simulink model "gm_Model"  (R2025a)
settings: Solver=FixedStepDiscrete  StartTime=0.0  StopTime=80000/fs_in  RelTol=1e-3
undefined symbols (not defined in the file or in its folder): a, b, b_fixp, beta_retanh, c, cos_omega, cos_omega_fixp, diag_count, exp_omega, exp_omega_fixp, fixp_chebacc_frac, fixp_chebacc_ws, fixp_dsp_ws, fixp_eig_frac, fixp_eig_ws, fs_in, group_size, hann_table_fixp, image_seed, image_seed_fixp, J_ROM, k, K_ROM, lap_diags, lap_main, lap_main_fi, lap_offsets, lap_offsets_fi, lap_rest, lap_rest_fi, laplacian_diags_main, laplacian_diags_offsets, laplacian_diags_rest, lut_norm_x, lut_norm_y, magnitude, n_ch, n_layer, n_px, n_px_fi, nf, norm_gain_floor, power_iters, power_norm_scaling_factor_fixp, tau, tau_fixp, theta, theta_fixp
libraries: simulink x59, hdlsllib x36, hdlstreaminglib x4, hdlmdlgenlib x1, matrix_library x1, dspvision x1
(part 2 of 8)

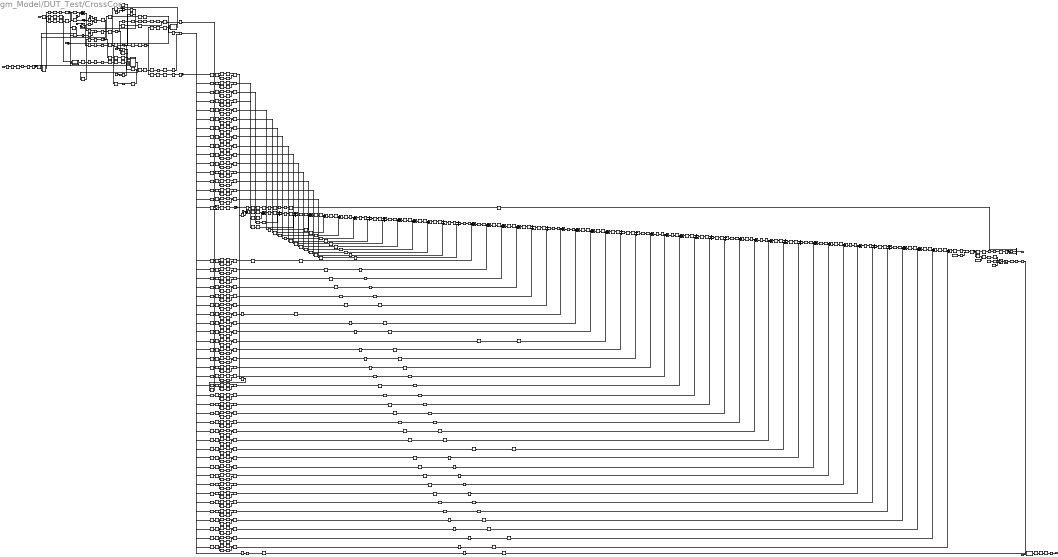
== system gm_Model/DUT_Test/CrossCor ==
  note: Sum 9 frames and reduce data rate
  valid_in : Inport  OutDataTypeStr=boolean  PortDimensions=1  SampleTime=0.0125
  data_in : Inport  Port=2  OutDataTypeStr=fixdt(1, 18, 13)  PortDimensions=[1 48]  SampleTime=0.0125
      settings: SignalType=complex
  sch_ctr_359999 : Inport  Port=3  OutDataTypeStr=fixdt(0, 19, 0)  SampleTime=3.125e-07
  sch_ctr_39999 : Inport  Port=4  OutDataTypeStr=uint16  SampleTime=3.125e-07
  AND : Logic  AllPortsSameDT=off  OutDataTypeStr=boolean  SampleTime=3.125e-07
  Bus Creator2 : BusCreator  Inputs=3
  Compare To Constant2 : simulink/Logic and Bit Operations/Compare To Constant  relop=<  const="fi(0,0,23,13,\"hex\",\"002000\")"  OutDataTypeStr=boolean
  Constant : Constant  Value=1.0001220703125  OutDataTypeStr=fixdt(0, 23, 13)  SampleTime=3.125e-07
  DataMem : RateTransition  InitialCondition=double(0)  OutPortSampleTimeOpt=Multiple of input port sample time  OutPortSampleTimeMultiple=40000
  DataMem_absorbed : Delay  DelayLength=0
  DataRT : RateTransition  InitialCondition=double(0)  OutPortSampleTimeOpt=Multiple of input port sample time  OutPortSampleTimeMultiple=9
  DataRT_outrepeat : RateTransition  Integrity=off  Deterministic=off  OutPortSampleTimeOpt=Multiple of input port sample time  OutPortSampleTimeMultiple=1/360000
  Delay{,1,7,11} (4 alike) : RateTransition  InitialCondition=double(0)  OutPortSampleTimeOpt=Multiple of input port sample time  OutPortSampleTimeMultiple=40000
  Delay1_absorbed{,1..3} (4 alike) : Delay  DelayLength=0
  Delay{2..6} (5 alike) : RateTransition  InitialCondition=double(0)  OutPortSampleTimeOpt=Multiple of input port sample time  OutPortSampleTimeMultiple=360000
  Delay2_absorbed : Delay  DelayLength=0
  Delay3_absorbed : Delay  DelayLength=0
  Delay4_absorbed : Delay  DelayLength=0
  Delay5_absorbed : Delay  DelayLength=0
  Delay6_absorbed : Delay  DelayLength=0
  Delay_Switch : Switch  Criteria=u2 ~= 0  Threshold=double(0)  OutDataTypeStr=boolean  SampleTime=3.125e-07  SaturateOnIntegerOverflow=off  InputSameDT=off
  Delay_absorbed : Delay  DelayLength=0
  Delay_absorbed1 : Delay  DelayLength=0
  Delay_absorbed2 : Delay  DelayLength=0
  Gain : Product  Inputs=**  OutDataTypeStr=fixdt(0, 23, 13)  SampleTime=3.125e-07
  Gain_const : Constant  Value=0.7071075439453125  OutDataTypeStr=fixdt(0, 18, 18)  SampleTime=3.125e-07
  HDL Counter : RateTransition  InitialCondition=double(0)  OutPortSampleTimeOpt=Multiple of input port sample time  OutPortSampleTimeMultiple=40000
  HDL Counter_absorbed : Delay  DelayLength=0
  HwModeRegister : Delay  DelayLength=double(1)  InitialCondition=0  SampleTime=3.125e-07
  HwModeRegister1 : Delay  DelayLength=double(1)  InitialCondition=0  SampleTime=3.125e-07
  Math Function1 : Math  Operator=hermitian  OutputSignalType=complex
  Max1_stage1 : MinMax  Function=max  Inputs=2
  NOT : Logic  Operator=NOT  Inputs=1  AllPortsSameDT=off  OutDataTypeStr=boolean  SampleTime=3.125e-07
  PipelineRegister : Delay  DelayLength=double(1)  InitialCondition=0  SampleTime=3.125e-07
  PipelineRegister1 : Delay  DelayLength=double(1)  InitialCondition=0  SampleTime=0.1125
  PipelineRegister2 : Delay  DelayLength=double(1)  InitialCondition=0  SampleTime=0.1125
  Real-Imag to Complex : RealImagToComplex  ConstantPart="fi(0,1,18,13,\"hex\",\"00000\")"  SampleTime=3.125e-07
  Real-Imag to Complex1 : RealImagToComplex  ConstantPart="fi(0,1,18,13,\"hex\",\"00000\")"  SampleTime=3.125e-07
  Reciprocal : Subsystem
  Row2Col_in0 : Reshape  OutputDimensionality=Column vector (2-D)
  Row2Col_in1 : Reshape  OutputDimensionality=Column vector (2-D)
  Selector : Selector  NumberOfDimensions=2  IndexOptions=Index vector (dialog),Index vector (dialog)  Indices=double(48),double(48)  OutputSizes=double(0),double(0)
  Selector1 : Selector  NumberOfDimensions=2  IndexOptions=Index vector (dialog),Index vector (dialog)  Indices=double(48),double(48)  OutputSizes=double(0),double(0)
  Selector10 : Selector  NumberOfDimensions=2  IndexOptions=Index vector (dialog),Index vector (dialog)  Indices=double(43),double(43)  OutputSizes=double(0),double(0)
  Selector11 : Selector  NumberOfDimensions=2  IndexOptions=Index vector (dialog),Index vector (dialog)  Indices=double(43),double(43)  OutputSizes=double(0),double(0)
  Selector12 : Selector  NumberOfDimensions=2  IndexOptions=Index vector (dialog),Index vector (dialog)  Indices=double(42),double(42)  OutputSizes=double(0),double(0)
  Selector13 : Selector  NumberOfDimensions=2  IndexOptions=Index vector (dialog),Index vector (dialog)  Indices=double(42),double(42)  OutputSizes=double(0),double(0)
  Selector14 : Selector  NumberOfDimensions=2  IndexOptions=Index vector (dialog),Index vector (dialog)  Indices=double(41),double(41)  OutputSizes=double(0),double(0)
  Selector15 : Selector  NumberOfDimensions=2  IndexOptions=Index vector (dialog),Index vector (dialog)  Indices=double(41),double(41)  OutputSizes=double(0),double(0)
  Selector16 : Selector  NumberOfDimensions=2  IndexOptions=Index vector (dialog),Index vector (dialog)  Indices=double(40),double(40)  OutputSizes=double(0),double(0)
  Selector17 : Selector  NumberOfDimensions=2  IndexOptions=Index vector (dialog),Index vector (dialog)  Indices=double(40),double(40)  OutputSizes=double(0),double(0)
  Selector18 : Selector  NumberOfDimensions=2  IndexOptions=Index vector (dialog),Index vector (dialog)  Indices=double(39),double(39)  OutputSizes=double(0),double(0)
  Selector19 : Selector  NumberOfDimensions=2  IndexOptions=Index vector (dialog),Index vector (dialog)  Indices=double(39),double(39)  OutputSizes=double(0),double(0)
  Selector2 : Selector  NumberOfDimensions=2  IndexOptions=Index vector (dialog),Index vector (dialog)  Indices=double(47),double(47)  OutputSizes=double(0),double(0)
  Selector20 : Selector  NumberOfDimensions=2  IndexOptions=Index vector (dialog),Index vector (dialog)  Indices=double(38),double(38)  OutputSizes=double(0),double(0)
  Selector21 : Selector  NumberOfDimensions=2  IndexOptions=Index vector (dialog),Index vector (dialog)  Indices=double(38),double(38)  OutputSizes=double(0),double(0)
  Selector22 : Selector  NumberOfDimensions=2  IndexOptions=Index vector (dialog),Index vector (dialog)  Indices=double(37),double(37)  OutputSizes=double(0),double(0)
  Selector23 : Selector  NumberOfDimensions=2  IndexOptions=Index vector (dialog),Index vector (dialog)  Indices=double(37),double(37)  OutputSizes=double(0),double(0)
  Selector24 : Selector  NumberOfDimensions=2  IndexOptions=Index vector (dialog),Index vector (dialog)  Indices=double(36),double(36)  OutputSizes=double(0),double(0)
  Selector25 : Selector  NumberOfDimensions=2  IndexOptions=Index vector (dialog),Index vector (dialog)  Indices=double(36),double(36)  OutputSizes=double(0),double(0)
  Selector26 : Selector  NumberOfDimensions=2  IndexOptions=Index vector (dialog),Index vector (dialog)  Indices=double(35),double(35)  OutputSizes=double(0),double(0)
  Selector27 : Selector  NumberOfDimensions=2  IndexOptions=Index vector (dialog),Index vector (dialog)  Indices=double(35),double(35)  OutputSizes=double(0),double(0)
  Selector28 : Selector  NumberOfDimensions=2  IndexOptions=Index vector (dialog),Index vector (dialog)  Indices=double(34),double(34)  OutputSizes=double(0),double(0)
  Selector29 : Selector  NumberOfDimensions=2  IndexOptions=Index vector (dialog),Index vector (dialog)  Indices=double(34),double(34)  OutputSizes=double(0),double(0)
  Selector3 : Selector  NumberOfDimensions=2  IndexOptions=Index vector (dialog),Index vector (dialog)  Indices=double(47),double(47)  OutputSizes=double(0),double(0)
  Selector30 : Selector  NumberOfDimensions=2  IndexOptions=Index vector (dialog),Index vector (dialog)  Indices=double(33),double(33)  OutputSizes=double(0),double(0)
  Selector31 : Selector  NumberOfDimensions=2  IndexOptions=Index vector (dialog),Index vector (dialog)  Indices=double(33),double(33)  OutputSizes=double(0),double(0)
  Selector32 : Selector  NumberOfDimensions=2  IndexOptions=Index vector (dialog),Index vector (dialog)  Indices=double(32),double(32)  OutputSizes=double(0),double(0)
  Selector33 : Selector  NumberOfDimensions=2  IndexOptions=Index vector (dialog),Index vector (dialog)  Indices=double(32),double(32)  OutputSizes=double(0),double(0)
  Selector34 : Selector  NumberOfDimensions=2  IndexOptions=Index vector (dialog),Index vector (dialog)  Indices=double(31),double(31)  OutputSizes=double(0),double(0)
  Selector35 : Selector  NumberOfDimensions=2  IndexOptions=Index vector (dialog),Index vector (dialog)  Indices=double(31),double(31)  OutputSizes=double(0),double(0)
  Selector36 : Selector  NumberOfDimensions=2  IndexOptions=Index vector (dialog),Index vector (dialog)  Indices=double(30),double(30)  OutputSizes=double(0),double(0)
  Selector37 : Selector  NumberOfDimensions=2  IndexOptions=Index vector (dialog),Index vector (dialog)  Indices=double(30),double(30)  OutputSizes=double(0),double(0)
  Selector38 : Selector  NumberOfDimensions=2  IndexOptions=Index vector (dialog),Index vector (dialog)  Indices=double(29),double(29)  OutputSizes=double(0),double(0)
  Selector39 : Selector  NumberOfDimensions=2  IndexOptions=Index vector (dialog),Index vector (dialog)  Indices=double(29),double(29)  OutputSizes=double(0),double(0)
  Selector4 : Selector  NumberOfDimensions=2  IndexOptions=Index vector (dialog),Index vector (dialog)  Indices=double(46),double(46)  OutputSizes=double(0),double(0)
  Selector40 : Selector  NumberOfDimensions=2  IndexOptions=Index vector (dialog),Index vector (dialog)  Indices=double(28),double(28)  OutputSizes=double(0),double(0)
  Selector41 : Selector  NumberOfDimensions=2  IndexOptions=Index vector (dialog),Index vector (dialog)  Indices=double(28),double(28)  OutputSizes=double(0),double(0)
  Selector42 : Selector  NumberOfDimensions=2  IndexOptions=Index vector (dialog),Index vector (dialog)  Indices=double(27),double(27)  OutputSizes=double(0),double(0)
  Selector43 : Selector  NumberOfDimensions=2  IndexOptions=Index vector (dialog),Index vector (dialog)  Indices=double(27),double(27)  OutputSizes=double(0),double(0)
  Selector44 : Selector  NumberOfDimensions=2  IndexOptions=Index vector (dialog),Index vector (dialog)  Indices=double(26),double(26)  OutputSizes=double(0),double(0)
  Selector45 : Selector  NumberOfDimensions=2  IndexOptions=Index vector (dialog),Index vector (dialog)  Indices=double(26),double(26)  OutputSizes=double(0),double(0)
  Selector46 : Selector  NumberOfDimensions=2  IndexOptions=Index vector (dialog),Index vector (dialog)  Indices=double(25),double(25)  OutputSizes=double(0),double(0)
  Selector47 : Selector  NumberOfDimensions=2  IndexOptions=Index vector (dialog),Index vector (dialog)  Indices=double(25),double(25)  OutputSizes=double(0),double(0)
  Selector48 : Selector  NumberOfDimensions=2  IndexOptions=Index vector (dialog),Index vector (dialog)  Indices=double(24),double(24)  OutputSizes=double(0),double(0)
  Selector49 : Selector  NumberOfDimensions=2  IndexOptions=Index vector (dialog),Index vector (dialog)  Indices=double(24),double(24)  OutputSizes=double(0),double(0)
  Selector5 : Selector  NumberOfDimensions=2  IndexOptions=Index vector (dialog),Index vector (dialog)  Indices=double(46),double(46)  OutputSizes=double(0),double(0)
  Selector50 : Selector  NumberOfDimensions=2  IndexOptions=Index vector (dialog),Index vector (dialog)  Indices=double(23),double(23)  OutputSizes=double(0),double(0)
  Selector51 : Selector  NumberOfDimensions=2  IndexOptions=Index vector (dialog),Index vector (dialog)  Indices=double(23),double(23)  OutputSizes=double(0),double(0)
  Selector52 : Selector  NumberOfDimensions=2  IndexOptions=Index vector (dialog),Index vector (dialog)  Indices=double(22),double(22)  OutputSizes=double(0),double(0)
  Selector53 : Selector  NumberOfDimensions=2  IndexOptions=Index vector (dialog),Index vector (dialog)  Indices=double(22),double(22)  OutputSizes=double(0),double(0)
  Selector54 : Selector  NumberOfDimensions=2  IndexOptions=Index vector (dialog),Index vector (dialog)  Indices=double(21),double(21)  OutputSizes=double(0),double(0)
  Selector55 : Selector  NumberOfDimensions=2  IndexOptions=Index vector (dialog),Index vector (dialog)  Indices=double(21),double(21)  OutputSizes=double(0),double(0)
  Selector56 : Selector  NumberOfDimensions=2  IndexOptions=Index vector (dialog),Index vector (dialog)  Indices=double(20),double(20)  OutputSizes=double(0),double(0)
  Selector57 : Selector  NumberOfDimensions=2  IndexOptions=Index vector (dialog),Index vector (dialog)  Indices=double(20),double(20)  OutputSizes=double(0),double(0)
  Selector58 : Selector  NumberOfDimensions=2  IndexOptions=Index vector (dialog),Index vector (dialog)  Indices=double(19),double(19)  OutputSizes=double(0),double(0)
  Selector59 : Selector  NumberOfDimensions=2  IndexOptions=Index vector (dialog),Index vector (dialog)  Indices=double(19),double(19)  OutputSizes=double(0),double(0)
  Selector6 : Selector  NumberOfDimensions=2  IndexOptions=Index vector (dialog),Index vector (dialog)  Indices=double(45),double(45)  OutputSizes=double(0),double(0)
  Selector60 : Selector  NumberOfDimensions=2  IndexOptions=Index vector (dialog),Index vector (dialog)  Indices=double(18),double(18)  OutputSizes=double(0),double(0)
  Selector61 : Selector  NumberOfDimensions=2  IndexOptions=Index vector (dialog),Index vector (dialog)  Indices=double(18),double(18)  OutputSizes=double(0),double(0)
  Selector62 : Selector  NumberOfDimensions=2  IndexOptions=Index vector (dialog),Index vector (dialog)  Indices=double(17),double(17)  OutputSizes=double(0),double(0)
  Selector63 : Selector  NumberOfDimensions=2  IndexOptions=Index vector (dialog),Index vector (dialog)  Indices=double(17),double(17)  OutputSizes=double(0),double(0)
  Selector64 : Selector  NumberOfDimensions=2  IndexOptions=Index vector (dialog),Index vector (dialog)  Indices=double(16),double(16)  OutputSizes=double(0),double(0)
  Selector65 : Selector  NumberOfDimensions=2  IndexOptions=Index vector (dialog),Index vector (dialog)  Indices=double(16),double(16)  OutputSizes=double(0),double(0)
  Selector66 : Selector  NumberOfDimensions=2  IndexOptions=Index vector (dialog),Index vector (dialog)  Indices=double(15),double(15)  OutputSizes=double(0),double(0)
  Selector67 : Selector  NumberOfDimensions=2  IndexOptions=Index vector (dialog),Index vector (dialog)  Indices=double(15),double(15)  OutputSizes=double(0),double(0)
  Selector68 : Selector  NumberOfDimensions=2  IndexOptions=Index vector (dialog),Index vector (dialog)  Indices=double(14),double(14)  OutputSizes=double(0),double(0)
  Selector69 : Selector  NumberOfDimensions=2  IndexOptions=Index vector (dialog),Index vector (dialog)  Indices=double(14),double(14)  OutputSizes=double(0),double(0)
  Selector7 : Selector  NumberOfDimensions=2  IndexOptions=Index vector (dialog),Index vector (dialog)  Indices=double(45),double(45)  OutputSizes=double(0),double(0)
  Selector70 : Selector  NumberOfDimensions=2  IndexOptions=Index vector (dialog),Index vector (dialog)  Indices=double(13),double(13)  OutputSizes=double(0),double(0)
  Selector71 : Selector  NumberOfDimensions=2  IndexOptions=Index vector (dialog),Index vector (dialog)  Indices=double(13),double(13)  OutputSizes=double(0),double(0)
  Selector72 : Selector  NumberOfDimensions=2  IndexOptions=Index vector (dialog),Index vector (dialog)  Indices=double(12),double(12)  OutputSizes=double(0),double(0)
  Selector73 : Selector  NumberOfDimensions=2  IndexOptions=Index vector (dialog),Index vector (dialog)  Indices=double(12),double(12)  OutputSizes=double(0),double(0)
  Selector74 : Selector  NumberOfDimensions=2  IndexOptions=Index vector (dialog),Index vector (dialog)  Indices=double(11),double(11)  OutputSizes=double(0),double(0)
  Selector75 : Selector  NumberOfDimensions=2  IndexOptions=Index vector (dialog),Index vector (dialog)  Indices=double(11),double(11)  OutputSizes=double(0),double(0)
  Selector76 : Selector  NumberOfDimensions=2  IndexOptions=Index vector (dialog),Index vector (dialog)  Indices=double(10),double(10)  OutputSizes=double(0),double(0)
  Selector77 : Selector  NumberOfDimensions=2  IndexOptions=Index vector (dialog),Index vector (dialog)  Indices=double(10),double(10)  OutputSizes=double(0),double(0)
  Selector78 : Selector  NumberOfDimensions=2  IndexOptions=Index vector (dialog),Index vector (dialog)  Indices=double(9),double(9)  OutputSizes=double(0),double(0)
  Selector79 : Selector  NumberOfDimensions=2  IndexOptions=Index vector (dialog),Index vector (dialog)  Indices=double(9),double(9)  OutputSizes=double(0),double(0)
  Selector8 : Selector  NumberOfDimensions=2  IndexOptions=Index vector (dialog),Index vector (dialog)  Indices=double(44),double(44)  OutputSizes=double(0),double(0)
  Selector80 : Selector  NumberOfDimensions=2  IndexOptions=Index vector (dialog),Index vector (dialog)  Indices=double(8),double(8)  OutputSizes=double(0),double(0)
  Selector81 : Selector  NumberOfDimensions=2  IndexOptions=Index vector (dialog),Index vector (dialog)  Indices=double(8),double(8)  OutputSizes=double(0),double(0)
  Selector82 : Selector  NumberOfDimensions=2  IndexOptions=Index vector (dialog),Index vector (dialog)  Indices=double(7),double(7)  OutputSizes=double(0),double(0)
  Selector83 : Selector  NumberOfDimensions=2  IndexOptions=Index vector (dialog),Index vector (dialog)  Indices=double(7),double(7)  OutputSizes=double(0),double(0)
  Selector84 : Selector  NumberOfDimensions=2  IndexOptions=Index vector (dialog),Index vector (dialog)  Indices=double(6),double(6)  OutputSizes=double(0),double(0)
  Selector85 : Selector  NumberOfDimensions=2  IndexOptions=Index vector (dialog),Index vector (dialog)  Indices=double(6),double(6)  OutputSizes=double(0),double(0)
  Selector86 : Selector  NumberOfDimensions=2  IndexOptions=Index vector (dialog),Index vector (dialog)  Indices=double(5),double(5)  OutputSizes=double(0),double(0)
  Selector87 : Selector  NumberOfDimensions=2  IndexOptions=Index vector (dialog),Index vector (dialog)  Indices=double(5),double(5)  OutputSizes=double(0),double(0)
  Selector88 : Selector  NumberOfDimensions=2  IndexOptions=Index vector (dialog),Index vector (dialog)  Indices=double(4),double(4)  OutputSizes=double(0),double(0)
  Selector89 : Selector  NumberOfDimensions=2  IndexOptions=Index vector (dialog),Index vector (dialog)  Indices=double(4),double(4)  OutputSizes=double(0),double(0)
  Selector9 : Selector  NumberOfDimensions=2  IndexOptions=Index vector (dialog),Index vector (dialog)  Indices=double(44),double(44)  OutputSizes=double(0),double(0)
  Selector90 : Selector  NumberOfDimensions=2  IndexOptions=Index vector (dialog),Index vector (dialog)  Indices=double(3),double(3)  OutputSizes=double(0),double(0)
  Selector91 : Selector  NumberOfDimensions=2  IndexOptions=Index vector (dialog),Index vector (dialog)  Indices=double(3),double(3)  OutputSizes=double(0),double(0)
  Selector92 : Selector  NumberOfDimensions=2  IndexOptions=Index vector (dialog),Index vector (dialog)  Indices=double(2),double(2)  OutputSizes=double(0),double(0)
  Selector93 : Selector  NumberOfDimensions=2  IndexOptions=Index vector (dialog),Index vector (dialog)  Indices=double(2),double(2)  OutputSizes=double(0),double(0)
  Selector94 : Selector  NumberOfDimensions=2  IndexOptions=Index vector (dialog),Index vector (dialog)  Indices=double(1),double(1)  OutputSizes=double(0),double(0)
  Selector95 : Selector  NumberOfDimensions=2  IndexOptions=Index vector (dialog),Index vector (dialog)  Indices=double(1),double(1)  OutputSizes=double(0),double(0)
  ValidMem_lowered : RateTransition  InitialCondition=double(0)  OutPortSampleTimeOpt=Multiple of input port sample time  OutPortSampleTimeMultiple=40000
  ValidMem_lowered_absorbed : Delay  DelayLength=0
  ValidRT : RateTransition  InitialCondition=double(0)  OutPortSampleTimeOpt=Multiple of input port sample time  OutPortSampleTimeMultiple=9
  ValidRT_outrepeat : RateTransition  Integrity=off  Deterministic=off  OutPortSampleTimeOpt=Multiple of input port sample time  OutPortSampleTimeMultiple=1/360000
  ValidResetCounter : RateTransition  InitialCondition=double(0)  OutPortSampleTimeOpt=Multiple of input port sample time  OutPortSampleTimeMultiple=40000
  ValidResetCounter_absorbed : Delay  DelayLength=0
  ValidResetDelay : RateTransition  InitialCondition=double(0)  OutPortSampleTimeOpt=Multiple of input port sample time  OutPortSampleTimeMultiple=40000
  ValidResetDelay_absorbed : Delay  DelayLength=0
  ValidSampleOR : Logic  Operator=OR  AllPortsSameDT=off  OutDataTypeStr=boolean  SampleTime=3.125e-07
  Zero : Constant  Value=0  OutDataTypeStr=fixdt(1, 18, 13)  SampleTime=3.125e-07
  Zero1 : Constant  Value=0  OutDataTypeStr=fixdt(1, 18, 13)  SampleTime=3.125e-07
  adder{,1..47} (48 alike) : Sum  OutDataTypeStr=fixdt(1, 25, 13)  AccumDataTypeStr=fixdt(1, 25, 13)  SampleTime=3.125e-07
  adder48 : Sum  OutDataTypeStr=fixdt(0, 4, 0)  AccumDataTypeStr=fixdt(0, 4, 0)  SampleTime=3.125e-07
  adder49 : Sum  OutDataTypeStr=fixdt(0, 4, 0)  AccumDataTypeStr=fixdt(0, 4, 0)  SampleTime=3.125e-07
  compare : simulink/Logic and Bit Operations/Compare To Constant  relop=>  const="fi(0,0,4,0,\"hex\",\"e\")"  OutDataTypeStr=boolean
  compare1 : simulink/Logic and Bit Operations/Compare To Constant  relop===  const="fi(0,0,4,0,\"hex\",\"8\")"  OutDataTypeStr=boolean
  compare2 : simulink/Logic and Bit Operations/Compare To Constant  relop=>  const="fi(0,0,4,0,\"hex\",\"e\")"  OutDataTypeStr=boolean
  compare3 : simulink/Logic and Bit Operations/Compare To Constant  relop===  const="fi(0,0,4,0,\"hex\",\"8\")"  OutDataTypeStr=boolean
  const : Constant  Value=0  VectorParams1D=off  OutDataTypeStr=fixdt(0, 23, 13)  SampleTime=3.125e-07
  countFrom : Constant  Value=0  VectorParams1D=off  OutDataTypeStr=fixdt(0, 4, 0)  SampleTime=3.125e-07
  countFrom1 : Constant  Value=0  VectorParams1D=off  OutDataTypeStr=fixdt(0, 4, 0)  SampleTime=3.125e-07
  cplx2reim{,1..47} (48 alike) : ComplexToRealImag  Output=Real  SampleTime=3.125e-07
  cplx2reim{48..95} (48 alike) : ComplexToRealImag  SampleTime=3.125e-07
  crp_out_delay{,1..11} (12 alike) : Delay  DelayLength=double(1)  InitialCondition=0  SampleTime=3.125e-07
  default_value : Constant  Value=fi(1,0,23,13)  OutDataTypeStr=fixdt(0, 23, 13)  SampleTime=3.125e-07
  delayMatch : Delay  DelayLength=double(40000)  InitialCondition=0  SampleTime=3.125e-07
  delayMatch1 : Delay  DelayLength=double(8)  InitialCondition=0  SampleTime=0.0125
  delayMatch2 : Delay  DelayLength=double(8)  InitialCondition=0  SampleTime=0.0125
  delayMatch3 : Delay  DelayLength=double(360000)  InitialCondition=0  SampleTime=3.125e-07
  delayMatch4 : Delay  DelayLength=double(360000)  InitialCondition=0  SampleTime=3.125e-07
  dtc{,1..47} (48 alike) : DataTypeConversion  OutDataTypeStr=fixdt(0, 23, 13)  SampleTime=3.125e-07  SaturateOnIntegerOverflow=off  RndMeth=Floor
  dtc48 : hdlmdlgenlib/Buffer
  in0_repeat : RateTransition  Integrity=off  Deterministic=off  OutPortSampleTimeOpt=Multiple of input port sample time  OutPortSampleTimeMultiple=1/40000
  in0_repeat1 : RateTransition  Integrity=off  Deterministic=off  OutPortSampleTimeOpt=Multiple of input port sample time  OutPortSampleTimeMultiple=1/40000
  in0_repeat2 : RateTransition  Integrity=off  Deterministic=off  OutPortSampleTimeOpt=Multiple of input port sample time  OutPortSampleTimeMultiple=1/360000
  in0_repeat3 : RateTransition  Integrity=off  Deterministic=off  OutPortSampleTimeOpt=Multiple of input port sample time  OutPortSampleTimeMultiple=1/40000
  in1_repeat : RateTransition  Integrity=off  Deterministic=off  OutPortSampleTimeOpt=Multiple of input port sample time  OutPortSampleTimeMultiple=1/40000
  in1_repeat1 : RateTransition  Integrity=off  Deterministic=off  OutPortSampleTimeOpt=Multiple of input port sample time  OutPortSampleTimeMultiple=1/360000
  in1_repeat2 : RateTransition  Integrity=off  Deterministic=off  OutPortSampleTimeOpt=Multiple of input port sample time  OutPortSampleTimeMultiple=1/40000
  in1_repeat3 : RateTransition  Integrity=off  Deterministic=off  OutPortSampleTimeOpt=Multiple of input port sample time  OutPortSampleTimeMultiple=1/40000
  in2_repeat : RateTransition  Integrity=off  Deterministic=off  OutPortSampleTimeOpt=Multiple of input port sample time  OutPortSampleTimeMultiple=1/40000
  in2_repeat1 : RateTransition  Integrity=off  Deterministic=off  OutPortSampleTimeOpt=Multiple of input port sample time  OutPortSampleTimeMultiple=1/360000
  in2_repeat2 : RateTransition  Integrity=off  Deterministic=off  OutPortSampleTimeOpt=Multiple of input port sample time  OutPortSampleTimeMultiple=1/40000
  in2_repeat3 : RateTransition  Integrity=off  Deterministic=off  OutPortSampleTimeOpt=Multiple of input port sample time  OutPortSampleTimeMultiple=1/40000
  in3_repeat : RateTransition  Integrity=off  Deterministic=off  OutPortSampleTimeOpt=Multiple of input port sample time  OutPortSampleTimeMultiple=1/40000
  in3_repeat1 : RateTransition  Integrity=off  Deterministic=off  OutPortSampleTimeOpt=Multiple of input port sample time  OutPortSampleTimeMultiple=1/360000
  in3_repeat2 : RateTransition  Integrity=off  Deterministic=off  OutPortSampleTimeOpt=Multiple of input port sample time  OutPortSampleTimeMultiple=1/40000
  in4_repeat : RateTransition  Integrity=off  Deterministic=off  OutPortSampleTimeOpt=Multiple of input port sample time  OutPortSampleTimeMultiple=1/40000
  in4_repeat1 : RateTransition  Integrity=off  Deterministic=off  OutPortSampleTimeOpt=Multiple of input port sample time  OutPortSampleTimeMultiple=1/40000
  in5_repeat : RateTransition  Integrity=off  Deterministic=off  OutPortSampleTimeOpt=Multiple of input port sample time  OutPortSampleTimeMultiple=1/40000
  or : Logic  Operator=OR  AllPortsSameDT=off  OutDataTypeStr=boolean  SampleTime=3.125e-07
  or1 : Logic  Operator=OR  AllPortsSameDT=off  OutDataTypeStr=boolean  SampleTime=3.125e-07
  rd_{0..4,6,8,10,12,14,16,18,20,22,24,26,28,30,32,34,36,38,40,42,44,46,48,50,52,54,56,58,60,62,64,66,68,70,72,74,76,78,80,82,84,86,88,90,92,94,96..98,101..102,110..112,121,131,141,210..212,310,411,510..511,610..612,710,810,910} (74 alike) : Delay  DelayLength=double(1)  InitialCondition=0  SampleTime=3.125e-07
  rd_01 : Delay  DelayLength=double(1)  InitialCondition=0  SampleTime=3.125e-07
  rd_02 : Delay  DelayLength=double(1)  InitialCondition=0  SampleTime=3.125e-07
  rd_03 : Delay  DelayLength=double(1)  InitialCondition=0  SampleTime=3.125e-07
  rd_04 : Delay  DelayLength=double(1)  InitialCondition=0  SampleTime=3.125e-07
  rd_103 : Delay  DelayLength=double(4)  InitialCondition=0  SampleTime=3.125e-07
  rd_11 : Delay  DelayLength=double(5)  InitialCondition=0  SampleTime=3.125e-07
  rd_13 : Delay  DelayLength=double(6)  InitialCondition=0  SampleTime=3.125e-07
  rd_15 : Delay  DelayLength=double(7)  InitialCondition=0  SampleTime=3.125e-07
  rd_17 : Delay  DelayLength=double(8)  InitialCondition=0  SampleTime=3.125e-07
  rd_19 : Delay  DelayLength=double(9)  InitialCondition=0  SampleTime=3.125e-07
  rd_21 : Delay  DelayLength=double(10)  InitialCondition=0  SampleTime=3.125e-07
  rd_23 : Delay  DelayLength=double(11)  InitialCondition=0  SampleTime=3.125e-07
  rd_25 : Delay  DelayLength=double(12)  InitialCondition=0  SampleTime=3.125e-07
  rd_27 : Delay  DelayLength=double(13)  InitialCondition=0  SampleTime=3.125e-07
  rd_29 : Delay  DelayLength=double(14)  InitialCondition=0  SampleTime=3.125e-07
  rd_31 : Delay  DelayLength=double(15)  InitialCondition=0  SampleTime=3.125e-07
  rd_{5,311,410,712} (4 alike) : Delay  DelayLength=double(2)  InitialCondition=0  SampleTime=3.125e-07
  rd_33 : Delay  DelayLength=double(16)  InitialCondition=0  SampleTime=3.125e-07
  rd_35 : Delay  DelayLength=double(17)  InitialCondition=0  SampleTime=3.125e-07
  rd_37 : Delay  DelayLength=double(18)  InitialCondition=0  SampleTime=3.125e-07
  rd_39 : Delay  DelayLength=double(19)  InitialCondition=0  SampleTime=3.125e-07
  rd_41 : Delay  DelayLength=double(20)  InitialCondition=0  SampleTime=3.125e-07
  rd_43 : Delay  DelayLength=double(21)  InitialCondition=0  SampleTime=3.125e-07
  rd_45 : Delay  DelayLength=double(22)  InitialCondition=0  SampleTime=3.125e-07
  rd_47 : Delay  DelayLength=double(23)  InitialCondition=0  SampleTime=3.125e-07
  rd_49 : Delay  DelayLength=double(24)  InitialCondition=0  SampleTime=3.125e-07
  rd_51 : Delay  DelayLength=double(25)  InitialCondition=0  SampleTime=3.125e-07
  rd_53 : Delay  DelayLength=double(26)  InitialCondition=0  SampleTime=3.125e-07
  rd_55 : Delay  DelayLength=double(27)  InitialCondition=0  SampleTime=3.125e-07
  rd_57 : Delay  DelayLength=double(28)  InitialCondition=0  SampleTime=3.125e-07
  rd_59 : Delay  DelayLength=double(29)  InitialCondition=0  SampleTime=3.125e-07
  rd_61 : Delay  DelayLength=double(30)  InitialCondition=0  SampleTime=3.125e-07
  rd_63 : Delay  DelayLength=double(31)  InitialCondition=0  SampleTime=3.125e-07
  rd_65 : Delay  DelayLength=double(32)  InitialCondition=0  SampleTime=3.125e-07
  rd_67 : Delay  DelayLength=double(33)  InitialCondition=0  SampleTime=3.125e-07
  rd_69 : Delay  DelayLength=double(34)  InitialCondition=0  SampleTime=3.125e-07
  rd_7 : Delay  DelayLength=double(3)  InitialCondition=0  SampleTime=3.125e-07
  rd_71 : Delay  DelayLength=double(35)  InitialCondition=0  SampleTime=3.125e-07
  rd_711 : Delay  DelayLength=double(3)  InitialCondition=0  SampleTime=3.125e-07
  rd_73 : Delay  DelayLength=double(36)  InitialCondition=0  SampleTime=3.125e-07
  rd_75 : Delay  DelayLength=double(37)  InitialCondition=0  SampleTime=3.125e-07
  rd_77 : Delay  DelayLength=double(38)  InitialCondition=0  SampleTime=3.125e-07
  rd_79 : Delay  DelayLength=double(39)  InitialCondition=0  SampleTime=3.125e-07
  rd_81 : Delay  DelayLength=double(40)  InitialCondition=0  SampleTime=3.125e-07
  rd_811 : Delay  DelayLength=double(3)  InitialCondition=0  SampleTime=3.125e-07
  rd_83 : Delay  DelayLength=double(41)  InitialCondition=0  SampleTime=3.125e-07
  rd_85 : Delay  DelayLength=double(42)  InitialCondition=0  SampleTime=3.125e-07
  rd_87 : Delay  DelayLength=double(43)  InitialCondition=0  SampleTime=3.125e-07
  rd_89 : Delay  DelayLength=double(44)  InitialCondition=0  SampleTime=3.125e-07
  rd_9 : Delay  DelayLength=double(4)  InitialCondition=0  SampleTime=3.125e-07
  rd_91 : Delay  DelayLength=double(45)  InitialCondition=0  SampleTime=3.125e-07
  rd_93 : Delay  DelayLength=double(46)  InitialCondition=0  SampleTime=3.125e-07
  rd_95 : Delay  DelayLength=double(47)  InitialCondition=0  SampleTime=3.125e-07
  rd_99 : Delay  DelayLength=double(51)  InitialCondition=0  SampleTime=3.125e-07
  reim2cplx{,1..47} (48 alike) : RealImagToComplex  ConstantPart="fi(0,1,18,13,\"hex\",\"00000\")"  SampleTime=3.125e-07
  reshape_mmulResult : Reshape  OutputDimensionality=Customize  OutputDimensions=[48,48]
  select_indices0 : Selector  InputPortWidth=48  IndexOptions=Index vector (dialog)  Indices=double([1;2;3;4;5;6;7;8;9;10;11;12;13;14;15;16;17;18;19;20;21;22;23;24;25;26;27;28;29;30;31;32;33;34;35;36;37;38;39;40;41;42;43;44;45;46;47;48;1;2;3;4;5;6;7;8;9;10;11;12;13;14;15;16;17;18;19;20;21;22;23;24;25;26;27;28;29;30;31;32;33;34;35;36;37;38;39;40;41;42;43;44;45;46;47;48;1;2;3;4;5;6;7;8;9;10;11;12;13;14;15;16;17;18;19;20;21;22;23;24;25;26;27;28;29;30;31;32;33;34;35;36;37;38;39;40;41;42;43;44;45;46;47;48;1;2;3;4;5;6;7;8;9;10;11;12;13;14;15;16;17;18;19;20;21;22;23;24;25;26;27;28;29;30;31;32;33;34;35;36;37;38;39;40;41;42;43;44;45;46;47;48;1;2;3;4;5;6;7;8;9;10;11;12;13;14;15;16;17;18;19;20;21;22;23;24;25;26;27;28;29;30;31;32;33;34;35;36;37;38;39;40;41;42;43;44;45;46;47;48;1;2;3;4;5;6;7;8;9;10;11;12;13;14;15;16;17;18;19;20;21;22;23;24;25;26;27;28;29;30;31;32;33;34;35;36;37;38;39;40;41;42;43;44;45;46;47;48;1;2;3;4;5;6;7;8;9;10;11;12;13;14;15;16;17;18;19;20;21;22;23;24;25;26;27;28;29;30;31;32;33;34;35;36;37;38;39;40;41;42;43;44;45;46;47;48;1;2;3;4;5;6;7;8;9;10;11;12;13;14;15;16;17;18;19;20;21;22;23;24;25;26;27;28;29;30;31;32;33;34;35;36;37;38;39;40;41;42;43;44;45;46;47;48;1;2;3;4;5;6;7;8;9;10;11;12;13;14;15;16;17;18;19;20;21;22;23;24;25;26;27;28;29;30;31;32;33;34;35;36;37;38;39;40;41;42;43;44;45;46;47;48;1;2;3;4;5;6;7;8;9;10;11;12;13;14;15;16;17;18;19;20;21;22;23;24;25;26;27;28;29;30;31;32;33;34;35;36;37;38;39;40;41;42;43;44;45;46;47;48;1;2;3;4;5;6;7;8;9;10;11;12;13;14;15;16;17;18;19;20;21;22;23;24;25;26;27;28;29;30;31;32;33;34;35;36;37;38;39;40;41;42;43;44;45;46;47;48;1;2;3;4;5;6;7;8;9;10;11;12;13;14;15;16;17;18;19;20;21;22;23;24;25;26;27;28;29;30;31;32;33;34;35;36;37;38;39;40;41;42;43;44;45;46;47;48;1;2;3;4;5;6;7;8;9;10;11;12;13;14;15;16;17;18;19;20;21;22;23;24;25;26;27;28;29;30;31;32;33;34;35;36;37;38;39;40;41;42;43;44;45;46;47;48;1;2;3;4;5;6;7;8;9;10;11;12;13;14;15;16;17;18;19;20;21;22;23;24;25;26;27;28;29;30;31;32;33;34;35;36;37;38;39;40;41;42;43;44;45;46;47;48;1;2;3;4;5;6;7;8;9;10;11;12;13;14;15;16;17;18;19;20;21;22;23;24;25;26;27;28;29;30;31;32;33;34;35;36;37;38;39;40;41;42;43;44;45;46;47;48;1;2;3;4;5;6;7;8;9;10;11;12;13;14;15;16;17;18;19;20;21;22;23;24;25;26;27;28;29;30;31;32;33;34;35;36;37;38;39;40;41;42;43;44;45;46;47;48;1;2;3;4;5;6;7;8;9;10;11;12;13;14;15;16;17;18;19;20;21;22;23;24;25;26;27;28;29;30;31;32;33;34;35;36;37;38;39;40;41;42;43;44;45;46;47;48;1;2;3;4;5;6;7;8;9;10;11;12;13;14;15;16;17;18;19;20;21;22;23;24;25;26;27;28;29;30;31;32;33;34;35;36;37;38;39;40;41;42;43;44;45;46;47;48;1;2;3;4;5;6;7;8;9;10;11;12;13;14;15;16;17;18;19;20;21;22;23;24;25;26;27;28;29;30;31;32;33;34;35;36;37;38;39;40;41;42;43;44;45;46;47;48;1;2;3;4;5;6;7;8;9;10;11;12;13;14;15;16;17;18;19;20;21;22;23;24;25;26;27;28;29;30;31;32;33;34;35;36;37;38;39;40;41;42;43;44;45;46;47;48;1;2;3;4;5;6;7;8;9;10;11;12;13;14;15;16;17;18;19;20;21;22;23;24;25;26;27;28;29;30;31;32;33;34;35;36;37;38;39;40;41;42;43;44;45;46;47;48;1;2;3;4;5;6;7;8;9;10;11;12;13;14;15;16;17;18;19;20;21;22;23;24;25;26;27;28;29;30;31;32;33;34;35;36;37;38;39;40;41;42;43;44;45;46;47;48;1;2;3;4;5;6;7;8;9;10;11;12;13;14;15;16;17;18;19;20;21;22;23;24;25;26;27;28;29;30;31;32;33;34;35;36;37;38;39;40;41;42;43;44;45;46;47;48;1;2;3;4;5;6;7;8;9;10;11;12;13;14;15;16;17;18;19;20;21;22;23;24;25;26;27;28;29;30;31;32;33;34;35;36;37;38;39;40;41;42;43;44;45;46;47;48;1;2;3;4;5;6;7;8;9;10;11;12;13;14;15;16;17;18;19;20;21;22;23;24;25;26;27;28;29;30;31;32;33;34;35;36;37;38;39;40;41;42;43;44;45;46;47;48;1;2;3;4;5;6;7;8;9;10;11;12;13;14;15;16;17;18;19;20;21;22;23;24;25;26;27;28;29;30;31;32;33;34;35;36;37;38;39;40;41;42;43;44;45;46;47;48;1;2;3;4;5;6;7;8;9;10;11;12;13;14;15;16;17;18;19;20;21;22;23;24;25;26;27;28;29;30;31;32;33;34;35;36;37;38;39;40;41;42;43;44;45;46;47;48;1;2;3;4;5;6;7;8;9;10;11;12;13;14;15;16;17;18;19;20;21;22;23;24;25;26;27;28;29;30;31;32;33;34;35;36;37;38;39;40;41;42;43;44;45;46;47;48;1;2;3;4;5;6;7;8;9;10;11;12;13;14;15;16;17;18;19;20;21;22;23;24;25;26;27;28;29;30;31;32;33;34;35;36;37;38;39;40;41;42;43;44;45;46;47;48;1;2;3;4;5;6;7;8;9;10;11;12;13;14;15;16;17;18;19;20;21;22;23;24;25;26;27;28;29;30;31 ...(+2481 chars)])  OutputSizes=1
  select_indices1 : Selector  InputPortWidth=48  IndexOptions=Index vector (dialog)  Indices=double([1;1;1;1;1;1;1;1;1;1;1;1;1;1;1;1;1;1;1;1;1;1;1;1;1;1;1;1;1;1;1;1;1;1;1;1;1;1;1;1;1;1;1;1;1;1;1;1;2;2;2;2;2;2;2;2;2;2;2;2;2;2;2;2;2;2;2;2;2;2;2;2;2;2;2;2;2;2;2;2;2;2;2;2;2;2;2;2;2;2;2;2;2;2;2;2;3;3;3;3;3;3;3;3;3;3;3;3;3;3;3;3;3;3;3;3;3;3;3;3;3;3;3;3;3;3;3;3;3;3;3;3;3;3;3;3;3;3;3;3;3;3;3;3;4;4;4;4;4;4;4;4;4;4;4;4;4;4;4;4;4;4;4;4;4;4;4;4;4;4;4;4;4;4;4;4;4;4;4;4;4;4;4;4;4;4;4;4;4;4;4;4;5;5;5;5;5;5;5;5;5;5;5;5;5;5;5;5;5;5;5;5;5;5;5;5;5;5;5;5;5;5;5;5;5;5;5;5;5;5;5;5;5;5;5;5;5;5;5;5;6;6;6;6;6;6;6;6;6;6;6;6;6;6;6;6;6;6;6;6;6;6;6;6;6;6;6;6;6;6;6;6;6;6;6;6;6;6;6;6;6;6;6;6;6;6;6;6;7;7;7;7;7;7;7;7;7;7;7;7;7;7;7;7;7;7;7;7;7;7;7;7;7;7;7;7;7;7;7;7;7;7;7;7;7;7;7;7;7;7;7;7;7;7;7;7;8;8;8;8;8;8;8;8;8;8;8;8;8;8;8;8;8;8;8;8;8;8;8;8;8;8;8;8;8;8;8;8;8;8;8;8;8;8;8;8;8;8;8;8;8;8;8;8;9;9;9;9;9;9;9;9;9;9;9;9;9;9;9;9;9;9;9;9;9;9;9;9;9;9;9;9;9;9;9;9;9;9;9;9;9;9;9;9;9;9;9;9;9;9;9;9;10;10;10;10;10;10;10;10;10;10;10;10;10;10;10;10;10;10;10;10;10;10;10;10;10;10;10;10;10;10;10;10;10;10;10;10;10;10;10;10;10;10;10;10;10;10;10;10;11;11;11;11;11;11;11;11;11;11;11;11;11;11;11;11;11;11;11;11;11;11;11;11;11;11;11;11;11;11;11;11;11;11;11;11;11;11;11;11;11;11;11;11;11;11;11;11;12;12;12;12;12;12;12;12;12;12;12;12;12;12;12;12;12;12;12;12;12;12;12;12;12;12;12;12;12;12;12;12;12;12;12;12;12;12;12;12;12;12;12;12;12;12;12;12;13;13;13;13;13;13;13;13;13;13;13;13;13;13;13;13;13;13;13;13;13;13;13;13;13;13;13;13;13;13;13;13;13;13;13;13;13;13;13;13;13;13;13;13;13;13;13;13;14;14;14;14;14;14;14;14;14;14;14;14;14;14;14;14;14;14;14;14;14;14;14;14;14;14;14;14;14;14;14;14;14;14;14;14;14;14;14;14;14;14;14;14;14;14;14;14;15;15;15;15;15;15;15;15;15;15;15;15;15;15;15;15;15;15;15;15;15;15;15;15;15;15;15;15;15;15;15;15;15;15;15;15;15;15;15;15;15;15;15;15;15;15;15;15;16;16;16;16;16;16;16;16;16;16;16;16;16;16;16;16;16;16;16;16;16;16;16;16;16;16;16;16;16;16;16;16;16;16;16;16;16;16;16;16;16;16;16;16;16;16;16;16;17;17;17;17;17;17;17;17;17;17;17;17;17;17;17;17;17;17;17;17;17;17;17;17;17;17;17;17;17;17;17;17;17;17;17;17;17;17;17;17;17;17;17;17;17;17;17;17;18;18;18;18;18;18;18;18;18;18;18;18;18;18;18;18;18;18;18;18;18;18;18;18;18;18;18;18;18;18;18;18;18;18;18;18;18;18;18;18;18;18;18;18;18;18;18;18;19;19;19;19;19;19;19;19;19;19;19;19;19;19;19;19;19;19;19;19;19;19;19;19;19;19;19;19;19;19;19;19;19;19;19;19;19;19;19;19;19;19;19;19;19;19;19;19;20;20;20;20;20;20;20;20;20;20;20;20;20;20;20;20;20;20;20;20;20;20;20;20;20;20;20;20;20;20;20;20;20;20;20;20;20;20;20;20;20;20;20;20;20;20;20;20;21;21;21;21;21;21;21;21;21;21;21;21;21;21;21;21;21;21;21;21;21;21;21;21;21;21;21;21;21;21;21;21;21;21;21;21;21;21;21;21;21;21;21;21;21;21;21;21;22;22;22;22;22;22;22;22;22;22;22;22;22;22;22;22;22;22;22;22;22;22;22;22;22;22;22;22;22;22;22;22;22;22;22;22;22;22;22;22;22;22;22;22;22;22;22;22;23;23;23;23;23;23;23;23;23;23;23;23;23;23;23;23;23;23;23;23;23;23;23;23;23;23;23;23;23;23;23;23;23;23;23;23;23;23;23;23;23;23;23;23;23;23;23;23;24;24;24;24;24;24;24;24;24;24;24;24;24;24;24;24;24;24;24;24;24;24;24;24;24;24;24;24;24;24;24;24;24;24;24;24;24;24;24;24;24;24;24;24;24;24;24;24;25;25;25;25;25;25;25;25;25;25;25;25;25;25;25;25;25;25;25;25;25;25;25;25;25;25;25;25;25;25;25;25;25;25;25;25;25;25;25;25;25;25;25;25;25;25;25;25;26;26;26;26;26;26;26;26;26;26;26;26;26;26;26;26;26;26;26;26;26;26;26;26;26;26;26;26;26;26;26;26;26;26;26;26;26;26;26;26;26;26;26;26;26;26;26;26;27;27;27;27;27;27;27;27;27;27;27;27;27;27;27;27;27;27;27;27;27;27;27;27;27;27;27;27;27;27;27;27;27;27;27;27;27;27;27;27;27;27;27;27;27;27;27;27;28;28;28;28;28;28;28;28;28;28;28;28;28;28;28;28;28;28;28;28;28;28;28;28;28;28;28;28;28;28;28;28;28;28;28;28;28;28;28;28;28;28;28;28;28;28;28;28;29;29;29;29;29;29;29;29;29;29;29;29;29;29;29;29;29;29;29;29;29;29;29;29;29;29;29;29;29;29;29;29;29;29;29;29;29;29;29;29;29;29;29;29;29;29;29;29;30;30;30;30;30;30;30;30;30;30;30;30;30;30;30;30;30;30;30;30;30;30;30;30;30;30;30;30;30;30;30;30;30;30;30;30;30;30;30;30;30;30;30;30;30;30;30;30;31;31;31;31;31;31;31;31;31;31;31;31;31;31;31;31;31;31;31;31;31;31;31;31;31;31;31;31;31;31;31;31;31;31;31;31;31 ...(+2481 chars)])  OutputSizes=1
  select_signal : Constant  Value=double(1)  OutDataTypeStr=boolean  SampleTime=3.125e-07
  step_value : Constant  VectorParams1D=off  OutDataTypeStr=fixdt(0, 4, 0)  SampleTime=3.125e-07
  step_value1 : Constant  VectorParams1D=off  OutDataTypeStr=fixdt(0, 4, 0)  SampleTime=3.125e-07
  streaming_partition_streamed : Subsystem
  streaming_partition_streamed1 : Subsystem
  streaming_partition_streamed2 : Subsystem
  streaming_partition_streamed3 : Subsystem
  switch : Switch  Criteria=u2 ~= 0  Threshold="fi(0,0,1,0,\"hex\",\"0\")"  OutDataTypeStr=fixdt(0, 4, 0)  SampleTime=3.125e-07  SaturateOnIntegerOverflow=off  InputSameDT=off
  switch1 : Switch  Criteria=u2 ~= 0  Threshold="fi(0,0,1,0,\"hex\",\"0\")"  OutDataTypeStr=fixdt(0, 4, 0)  SampleTime=3.125e-07  SaturateOnIntegerOverflow=off  InputSameDT=off
  switchEnable : MultiPortSwitch  DataPortOrder=Zero-based contiguous  Inputs=2  DiagnosticForDefault=None  zeroidx=on  OutDataTypeStr=fixdt(0, 4, 0)  SampleTime=3.125e-07  SaturateOnIntegerOverflow=off  InputSameDT=off
  t{,2,5,8,11,14,17,20,23,26,29,32,35,38,41,44,47,50,53,56,59,62,65,68,71,74,77,80,83,86,89,92,95,98,101,104,107,110,113,116,119,122,125,128,131,134,137,140,143,146..147,149..150} (53 alike) : Reshape  OutputDimensionality=Column vector (2-D)
  t{1,3..4,6..7,9..10,12..13,15..16,18..19,21..22,24..25,27..28,30..31,33..34,36..37,39..40,42..43,45..46,48..49,51..52,54..55,57..58,60..61,63..64,66..67,69..70,72..73,75..76,78..79,81..82,84..85,87..88,90..91,93..94,96..97,99..100,102..103,105..106,108..109,111..112,114..115,117..118,120..121,123..124,126..127,129..130,132..133,135..136,138..139,141..142,144..145,148,151} (99 alike) : Reshape  OutputDimensionality=Customize  OutputDimensions=[48,48]
  zero_protection : Switch  Criteria=u2 ~= 0  Threshold=double(0)  OutDataTypeStr=fixdt(0, 23, 13)  SampleTime=3.125e-07  SaturateOnIntegerOverflow=off  InputSameDT=off
  status : Outport
  data_out : Outport  Port=2  SampleTime=0.1125
  wires:
  adder29/1 -> dtc29/1
  rd_26/1 -> adder34/1
  cplx2reim92/1 -> t138/1
  rd_411/1 -> t150/1
  dtc14/1 -> rd_68/1
  adder3/1 -> dtc3/1
  Selector/1 -> reim2cplx/2
  t8/1 -> cplx2reim49/1
  Gain/1 -> PipelineRegister/1
  Selector89/1 -> reim2cplx44/1
  reim2cplx7/1 -> cplx2reim7/1
  reim2cplx17/1 -> cplx2reim17/1
  rd_1/1 -> adder48/1
  cplx2reim82/1 -> t108/1
  t30/1 -> Selector19/1
  adder45/1 -> dtc45/1
  HwModeRegister1/1 -> Gain/2
  DataRT_outrepeat/1 -> rd_01/1
  cplx2reim82/2 -> t109/1
  Selector17/1 -> reim2cplx8/1
  Delay2_absorbed/1 -> data_out/1
  adder33/1 -> dtc33/1
  cplx2reim90/2 -> t133/1
  select_indices1/1 -> Row2Col_in1/1
  cplx2reim50/1 -> t12/1
  rd_111/1 -> Math Function1/1
  Selector64/1 -> reim2cplx32/2
  t51/1 -> Selector33/1
  rd_18/1 -> adder38/1
  streaming_partition_streamed/1(out0) -> t1/1
  t143/1 -> cplx2reim94/1
  cplx2reim23/1 -> rd_49/1
  t63/1 -> Selector41/1
  rd_910/1 -> Delay_Switch/2
  cplx2reim80/2 -> t103/1
  Real-Imag to Complex1/1 -> streaming_partition_streamed2/6(in5)
  Selector41/1 -> reim2cplx20/1
  t101/1 -> cplx2reim80/1
  cplx2reim38/1 -> rd_19/1
  DataRT/1 -> PipelineRegister1/1
  t102/1 -> Selector67/1
  ValidRT/1 -> PipelineRegister2/1
  cplx2reim86/2 -> t121/1
  t38/1 -> cplx2reim59/1
  rd_42/1 -> adder26/1
  rd_112/1 -> NOT/1
  cplx2reim61/2 -> t46/1
  HwModeRegister/1 -> Gain/1
  rd_141/1 -> or1/2
  t9/1 -> Selector5/1
  rd_3/1 -> adder46/2
  reshape_mmulResult/1 -> crp_out_delay6/1
  t5/1 -> cplx2reim48/1
  dtc32/1 -> rd_32/1
  rd_64/1 -> adder15/1
  t48/1 -> Selector31/1
  adder15/1 -> dtc15/1
  Max1_stage1/1 -> dtc48/1
  compare2/1 -> rd_141/1
  cplx2reim41/1 -> rd_13/1
  t136/1 -> Selector88/1
  rd_511/1 -> compare3/1
  t105/1 -> Selector69/1
  rd_22/1 -> adder36/1
  Selector63/1 -> reim2cplx31/1
  Selector94/1 -> reim2cplx47/2
  reim2cplx47/1 -> cplx2reim47/1
  rd_510/1 -> or/1
  t92/1 -> cplx2reim77/1
  crp_out_delay7/1 -> Delay7/1
  cplx2reim67/2 -> t64/1
  adder17/1 -> dtc17/1
  t86/1 -> cplx2reim75/1
  switchEnable/1 -> crp_out_delay8/1
  dtc5/1 -> rd_86/1
  rd_74/1 -> adder10/1
  or1/1 -> crp_out_delay9/1
  ValidMem_lowered/1 -> ValidMem_lowered_absorbed/1
  dtc47/1 -> rd_2/1
  Delay1/1 -> Delay1_absorbed/1
  rd_44/1 -> adder25/1
  rd_811/1 -> ValidSampleOR/2
  crp_out_delay3/1 -> ValidResetCounter/1
  cplx2reim91/1 -> t135/1
  adder11/1 -> dtc11/1
  PipelineRegister2/1 -> ValidRT_outrepeat/1
  in0_repeat3/1 -> rd_1/1, rd_610/1, rd_02/1
  Selector68/1 -> reim2cplx34/2
  zero_protection/1 -> Reciprocal/1(In1)
  dtc28/1 -> rd_40/1
  reim2cplx33/1 -> cplx2reim33/1
  ValidMem_lowered_absorbed/1 -> delayMatch2/1, in2_repeat3/1
  cplx2reim57/1 -> t33/1
  t17/1 -> cplx2reim52/1
  reim2cplx32/1 -> cplx2reim32/1
  rd_82/1 -> adder6/1
  t68/1 -> cplx2reim69/1
  t138/1 -> Selector91/1
  dtc34/1 -> rd_28/1
  Selector30/1 -> reim2cplx15/2
  default_value/1 -> zero_protection/3
  t36/1 -> Selector23/1
  rd_70/1 -> adder12/1
  dtc31/1 -> rd_34/1
  cplx2reim11/1 -> rd_73/1
  t24/1 -> Selector15/1
  sch_ctr_359999/1 -> streaming_partition_streamed/3(enb_counter)
  HDL Counter/1 -> HDL Counter_absorbed/1
  Selector51/1 -> reim2cplx25/1
  t57/1 -> Selector37/1
  cplx2reim69/2 -> t70/1
  Selector7/1 -> reim2cplx3/1
  t81/1 -> Selector53/1
  Bus Creator2/1 -> status/1
  cplx2reim59/2 -> t40/1
  rd_110/1 -> t146/1
  rd_612/1 -> ValidSampleOR/1
  t144/1 -> Selector95/1
  adder21/1 -> dtc21/1
  rd_103/1 -> Delay_Switch/3
  ValidResetDelay/1 -> ValidResetDelay_absorbed/1
  cplx2reim37/1 -> rd_21/1
  cplx2reim60/2 -> t43/1
  rd_76/1 -> adder9/1
  step_value1/1 -> adder49/2
  rd_51/1 -> adder22/2
  rd_212/1 -> AND/1
  rd_04/1 -> t149/1
  cplx2reim2/1 -> rd_91/1
  adder43/1 -> dtc43/1
  crp_out_delay4/1 -> ValidResetDelay/1
  rd_311/1 -> AND/2
  t100/1 -> Selector64/1
  rd_78/1 -> adder8/1
  NOT/1 -> rd_212/1
  t130/1 -> Selector84/1
  cplx2reim43/1 -> rd_9/1
  Selector4/1 -> reim2cplx2/2
  cplx2reim81/1 -> t105/1
  Selector86/1 -> reim2cplx43/2
  t150/1 -> streaming_partition_streamed3/3(in2)
  Selector28/1 -> reim2cplx14/2
  adder4/1 -> dtc4/1
  reim2cplx/1 -> cplx2reim/1
  Selector65/1 -> reim2cplx32/1
  t53/1 -> cplx2reim64/1
  t114/1 -> Selector75/1
  adder49/1 -> rd_96/1
  cplx2reim55/1 -> t27/1
  Delay_absorbed2/1 -> in2_repeat1/1
  reim2cplx26/1 -> cplx2reim26/1
  rd_68/1 -> adder13/1
  dtc12/1 -> rd_72/1
  Delay5_absorbed/1 -> in1_repeat1/1
  countFrom1/1 -> switch1/1
  cplx2reim72/2 -> t79/1
  rd_86/1 -> adder4/1
  rd_01/1 -> Delay4/1, t143/1, t140/1, t122/1, t119/1, t113/1, t110/1, t98/1, t95/1, t92/1, t86/1, t83/1, t77/1, t74/1, t71/1, t62/1, t59/1, t56/1, t47/1, t44/1, t41/1, t38/1, t35/1, t32/1, t29/1, t26/1, t23/1, t17/1, t14/1, t5/1, t2/1, t128/1, t125/1, t53/1, t8/1, t107/1, t89/1, t80/1, t68/1, t137/1, t101/1, t20/1, t116/1, t65/1, t104/1, t131/1, t50/1, t11/1, t134/1
  cplx2reim26/1 -> rd_43/1
  cplx2reim92/2 -> t139/1
  rd_810/1 -> switch1/2
  Real-Imag to Complex/1 -> streaming_partition_streamed2/1(in0)
  t41/1 -> cplx2reim60/1
  dtc48/1 -> rd_98/1
  cplx2reim91/2 -> t136/1
  rd_121/1 -> or1/1
  t127/1 -> Selector82/1
  t151/1 -> crp_out_delay10/1
  cplx2reim48/2 -> t7/1
  rd_46/1 -> adder24/1
  dtc2/1 -> rd_92/1
  Selector58/1 -> reim2cplx29/2
  t118/1 -> Selector76/1
  t22/1 -> Selector12/1
  t54/1 -> Selector35/1
  Delay_Switch/1 -> crp_out_delay11/1
  crp_out_delay5/1 -> Delay1/1
  cplx2reim77/1 -> t93/1
  Selector26/1 -> reim2cplx13/2
  t16/1 -> Selector8/1
  rd_5/1 -> adder45/2
  t82/1 -> Selector52/1
  DataMem_absorbed/1 -> in5_repeat/1, delayMatch1/1
  select_indices0/1 -> Row2Col_in0/1
  PipelineRegister/1 -> rd_97/1, crp_out_delay1/1
  ValidSampleOR/1 -> rd_910/1
  t83/1 -> cplx2reim74/1
  delayMatch4/1 -> Bus Creator2/3, Compare To Constant2/1  "norm"
  cplx2reim89/2 -> t130/1
  rd_38/1 -> adder28/1
  cplx2reim/1 -> rd_95/1
  t147/1 -> streaming_partition_streamed2/3(in2)
  t112/1 -> Selector72/1
  rd_60/1 -> adder17/1
  reim2cplx12/1 -> cplx2reim12/1
  rd_410/1 -> switchEnable/1
  Delay7/1 -> Delay_absorbed1/1
  delayMatch/1 -> rd_112/1
  adder41/1 -> dtc41/1
  Selector25/1 -> reim2cplx12/1
  adder47/1 -> dtc47/1
  t125/1 -> cplx2reim88/1
  Selector55/1 -> reim2cplx27/1
  dtc46/1 -> rd_4/1
  Delay6_absorbed/1 -> Delay1_absorbed2/1
  Selector67/1 -> reim2cplx33/1
  rd_96/1 -> switch1/3
  cplx2reim49/1 -> t9/1
  t33/1 -> Selector21/1
  Selector84/1 -> reim2cplx42/2
  Math Function1/1 -> select_indices0/1
  Row2Col_in0/1 -> streaming_partition_streamed1/2(in1)
  cplx2reim72/1 -> t78/1
  rd_03/1 -> t147/1
  t90/1 -> Selector59/1
  t132/1 -> Selector87/1
  rd_611/1 -> adder49/1
  t2/1 -> cplx2reim95/1
  reim2cplx4/1 -> cplx2reim4/1
  Selector70/1 -> reim2cplx35/2
  t89/1 -> cplx2reim76/1
  rd_211/1 -> streaming_partition_streamed2/5(in4), rd_410/1
  rd_131/1 -> compare2/1
  t146/1 -> streaming_partition_streamed2/4(in3)
  t61/1 -> Selector38/1
  cplx2reim63/2 -> t52/1
  adder20/1 -> dtc20/1
  rd_19/1 -> adder38/2
  t148/1 -> crp_out_delay7/1
  switch1/1 -> rd_102/1
  crp_out_delay/1 -> Delay2/1
  adder37/1 -> dtc37/1
  t91/1 -> Selector58/1
  rd_02/1 -> compare1/1
  t21/1 -> Selector13/1
  cplx2reim88/2 -> t127/1
  rd_92/1 -> adder1/1
  t73/1 -> Selector46/1
  cplx2reim93/1 -> t141/1
  cplx2reim49/2 -> t10/1
  rd_610/1 -> compare/1
  rd_23/1 -> adder36/2
  Selector85/1 -> reim2cplx42/1
  cplx2reim94/2 -> t145/1
  Delay3_absorbed/1 -> Delay_absorbed2/1
  rd_101/1 -> select_indices1/1
  rd_710/1 -> or/2
  streaming_partition_streamed1/1(out0) -> reshape_mmulResult/1
  Selector72/1 -> reim2cplx36/2
  dtc29/1 -> rd_38/1
  Selector91/1 -> reim2cplx45/1
  dtc17/1 -> rd_62/1
  t78/1 -> Selector51/1
  adder24/1 -> dtc24/1
  rd_31/1 -> adder32/2
  reim2cplx24/1 -> cplx2reim24/1
  cplx2reim53/2 -> t22/1
  crp_out_delay10/1 -> DataMem/1
  cplx2reim29/1 -> rd_37/1
  t120/1 -> Selector79/1
  Compare To Constant2/1 -> Bus Creator2/2  "norm_floor_hit"
  Selector33/1 -> reim2cplx16/1
  reim2cplx43/1 -> cplx2reim43/1
  rd_94/1 -> adder/1
  step_value/1 -> adder48/2
  adder48/1 -> rd_310/1
  switch/1 -> crp_out_delay3/1
  rd_52/1 -> adder21/1
  dtc42/1 -> rd_12/1
  adder34/1 -> dtc34/1
  or/1 -> crp_out_delay4/1
  cplx2reim81/2 -> t106/1
  cplx2reim27/1 -> rd_41/1
  compare/1 -> rd_710/1
  reim2cplx18/1 -> cplx2reim18/1
  cplx2reim54/2 -> t25/1
  t4/1 -> Selector/1
  countFrom/1 -> switch/1
  t11/1 -> cplx2reim50/1
  Selector39/1 -> reim2cplx19/1
  rd_83/1 -> adder6/2
  Selector50/1 -> reim2cplx25/2
  cplx2reim70/2 -> t73/1
  rd_72/1 -> adder11/1
  t20/1 -> cplx2reim53/1
  t106/1 -> Selector68/1
  Selector16/1 -> reim2cplx8/2
  t28/1 -> Selector16/1
  cplx2reim73/1 -> t81/1
  t135/1 -> Selector89/1
  rd_12/1 -> adder41/1
  crp_out_delay9/1 -> Delay11/1
  rd_80/1 -> adder7/1
  dtc41/1 -> rd_14/1
  t129/1 -> Selector85/1
  dtc25/1 -> rd_46/1
  cplx2reim65/2 -> t58/1
  rd_99/1 -> zero_protection/2
  rd_84/1 -> adder5/1
  crp_out_delay6/1 -> Delay/1
  t98/1 -> cplx2reim79/1
  rd_97/1 -> Max1_stage1/1
  Reciprocal/1(Out1) -> Delay5/1
  sch_ctr_39999/1 -> streaming_partition_streamed3/4(enb_counter), streaming_partition_streamed1/3(enb_counter), streaming_partition_streamed2/7(enb_counter)
  adder44/1 -> dtc44/1
  cplx2reim32/1 -> rd_31/1
  rd_98/1 -> zero_protection/1
  Selector1/1 -> reim2cplx/1
  cplx2reim68/1 -> t66/1
  Selector31/1 -> reim2cplx15/1
  cplx2reim54/1 -> t24/1
  rd_88/1 -> adder3/1
  rd_85/1 -> adder5/2
  t12/1 -> Selector7/1
  Selector23/1 -> reim2cplx11/1
  data_in/1 -> in2_repeat2/1
  rd_2/1 -> adder46/1
  Selector29/1 -> reim2cplx14/1
  t19/1 -> Selector10/1
  cplx2reim66/1 -> t60/1
  cplx2reim77/2 -> t94/1
  Delay1_absorbed2/1 -> in3_repeat1/1
  Selector19/1 -> reim2cplx9/1
  rd_4/1 -> adder45/1
  Selector57/1 -> reim2cplx28/1
  cplx2reim65/1 -> t57/1
  adder30/1 -> dtc30/1
  t74/1 -> cplx2reim71/1
  rd_6/1 -> adder44/1
  t50/1 -> cplx2reim63/1
  HDL Counter_absorbed/1 -> in1_repeat3/1
  rd_36/1 -> adder29/1
  rd_8/1 -> adder43/1
  t115/1 -> Selector74/1
  rd_9/1 -> adder43/2
  Selector52/1 -> reim2cplx26/2
  rd_66/1 -> adder14/1
  rd_10/1 -> adder42/1
  in1_repeat3/1 -> rd_611/1, rd_511/1, rd_711/1, rd_131/1
  cplx2reim71/1 -> t75/1
  Selector27/1 -> reim2cplx13/1
  t85/1 -> Selector54/1
  t70/1 -> Selector44/1
  dtc23/1 -> rd_50/1
  rd_90/1 -> adder2/1
  reim2cplx16/1 -> cplx2reim16/1
  t27/1 -> Selector17/1
  cplx2reim88/1 -> t126/1
  t47/1 -> cplx2reim62/1
  Selector76/1 -> reim2cplx38/2
  in2_repeat1/1 -> delayMatch3/1
  t133/1 -> Selector86/1
  cplx2reim63/1 -> t51/1
  adder8/1 -> dtc8/1
  rd_14/1 -> adder40/1
  rd_16/1 -> adder39/1
  cplx2reim83/2 -> t112/1
  delayMatch1/1 -> DataRT/1
  dtc43/1 -> rd_10/1
  cplx2reim84/1 -> t114/1
  cplx2reim31/1 -> rd_33/1
  ValidResetDelay_absorbed/1 -> in1_repeat/1
  rd_20/1 -> adder37/1
  t42/1 -> Selector27/1
  Selector61/1 -> reim2cplx30/1
  cplx2reim57/2 -> t34/1
  rd_24/1 -> adder35/1
  cplx2reim46/1 -> rd_3/1
  t35/1 -> cplx2reim58/1
  rd_28/1 -> adder33/1
  cplx2reim51/1 -> t15/1
  Selector92/1 -> reim2cplx46/2
  t107/1 -> cplx2reim82/1
  rd_30/1 -> adder32/1
  Selector43/1 -> reim2cplx21/1
  cplx2reim53/1 -> t21/1
  in2_repeat/1 -> rd_211/1
  rd_32/1 -> adder31/1
  rd_34/1 -> adder30/1
  Selector34/1 -> reim2cplx17/2
  rd_40/1 -> adder27/1
  reim2cplx20/1 -> cplx2reim20/1
  cplx2reim78/1 -> t96/1
  cplx2reim20/1 -> rd_55/1
  cplx2reim75/1 -> t87/1
  Selector2/1 -> reim2cplx1/2
  t124/1 -> Selector80/1
  cplx2reim75/2 -> t88/1
  Delay2/1 -> Delay2_absorbed/1
  Selector3/1 -> reim2cplx1/1
  rd_48/1 -> adder23/1
  cplx2reim74/1 -> t84/1
  t/1 -> streaming_partition_streamed/2(in1)
  t109/1 -> Selector70/1
  Selector48/1 -> reim2cplx24/2
  Selector37/1 -> reim2cplx18/1
  rd_50/1 -> adder22/1
  t96/1 -> Selector63/1
  cplx2reim45/1 -> rd_5/1
  adder25/1 -> dtc25/1
  t71/1 -> cplx2reim70/1
  cplx2reim76/1 -> t90/1
  cplx2reim85/1 -> t117/1
  Selector90/1 -> reim2cplx45/2
  Delay_absorbed1/1 -> in4_repeat1/1, in0_repeat1/1
  t140/1 -> cplx2reim93/1
  adder14/1 -> dtc14/1
  cplx2reim28/1 -> rd_39/1
  Selector87/1 -> reim2cplx43/1
  rd_54/1 -> adder20/1
  t103/1 -> Selector66/1
  Selector35/1 -> reim2cplx17/1
  cplx2reim78/2 -> t97/1
  rd_56/1 -> adder19/1
  dtc19/1 -> rd_58/1
  rd_58/1 -> adder18/1
  rd_61/1 -> adder17/2
  t77/1 -> cplx2reim72/1
  adder38/1 -> dtc38/1
  Delay3/1 -> Delay3_absorbed/1
  cplx2reim44/1 -> rd_7/1
  cplx2reim86/1 -> t120/1
  rd_62/1 -> adder16/1
  Selector11/1 -> reim2cplx5/1
  dtc13/1 -> rd_70/1
  t15/1 -> Selector9/1
  select_signal/1 -> rd_99/1
  cplx2reim55/2 -> t28/1
  Selector80/1 -> reim2cplx40/2
  t52/1 -> Selector32/1
  Gain_const/1 -> HwModeRegister1/1
  cplx2reim94/1 -> t144/1
  adder35/1 -> dtc35/1
  cplx2reim93/2 -> t142/1
  Delay1_absorbed/1 -> in2_repeat/1
  t137/1 -> cplx2reim92/1
  t123/1 -> Selector81/1
  Selector81/1 -> reim2cplx40/1
  t134/1 -> cplx2reim91/1
  cplx2reim90/1 -> t132/1
  compare3/1 -> rd_810/1, rd_121/1
  adder6/1 -> dtc6/1
  t131/1 -> cplx2reim90/1
  rd_67/1 -> adder14/2
  Selector32/1 -> reim2cplx16/2
  cplx2reim89/1 -> t129/1
  t128/1 -> cplx2reim89/1
  cplx2reim87/2 -> t124/1
  dtc27/1 -> rd_42/1
  cplx2reim87/1 -> t123/1
  t122/1 -> cplx2reim87/1
  t45/1 -> Selector29/1
  t13/1 -> Selector6/1
  t119/1 -> cplx2reim86/1
  Selector59/1 -> reim2cplx29/1
  cplx2reim85/2 -> t118/1
  cplx2reim60/1 -> t42/1
  t25/1 -> Selector14/1
  t116/1 -> cplx2reim85/1
  const/1 -> adder47/1
  Selector62/1 -> reim2cplx31/2
  adder23/1 -> dtc23/1
  cplx2reim84/2 -> t115/1
  t113/1 -> cplx2reim84/1
  dtc39/1 -> rd_18/1
  dtc24/1 -> rd_48/1
  Selector60/1 -> reim2cplx30/2
  cplx2reim58/2 -> t37/1
  cplx2reim83/1 -> t111/1
  dtc8/1 -> rd_80/1
  t110/1 -> cplx2reim83/1
  cplx2reim95/1 -> t3/1
  AND/1 -> rd_712/1, streaming_partition_streamed3/2(in1), rd_612/1
  dtc30/1 -> rd_36/1
  t32/1 -> cplx2reim57/1
  ValidResetCounter_absorbed/1 -> in0_repeat3/1
  t104/1 -> cplx2reim81/1
  rd_71/1 -> adder12/2
  cplx2reim80/1 -> t102/1
  cplx2reim79/2 -> t100/1
  Selector69/1 -> reim2cplx34/1
  cplx2reim79/1 -> t99/1
  cplx2reim48/1 -> t6/1
  Selector38/1 -> reim2cplx19/2
  Delay6/1 -> Delay6_absorbed/1
  t95/1 -> cplx2reim78/1
  rd_45/1 -> adder25/2
  cplx2reim76/2 -> t91/1
  cplx2reim56/1 -> t30/1
  t26/1 -> cplx2reim55/1
  cplx2reim74/2 -> t85/1
  cplx2reim95/2 -> t4/1
  adder16/1 -> dtc16/1
  in1_repeat2/1 -> crp_out_delay5/1
  cplx2reim73/2 -> t82/1
  t80/1 -> cplx2reim73/1
  Selector15/1 -> reim2cplx7/1
  cplx2reim71/2 -> t76/1
  cplx2reim70/1 -> t72/1
  cplx2reim69/1 -> t69/1
  cplx2reim68/2 -> t67/1
  Selector77/1 -> reim2cplx38/1
  Selector36/1 -> reim2cplx18/2
  t65/1 -> cplx2reim68/1
  cplx2reim61/1 -> t45/1
  cplx2reim67/1 -> t63/1
  t62/1 -> cplx2reim67/1
  cplx2reim66/2 -> t61/1
  t56/1 -> cplx2reim65/1
  t59/1 -> cplx2reim66/1
  rd_89/1 -> adder3/2
  cplx2reim64/2 -> t55/1
  adder42/1 -> dtc42/1
  cplx2reim64/1 -> t54/1
  in0_repeat1/1 -> rd_04/1
  adder46/1 -> dtc46/1
  Selector82/1 -> reim2cplx41/2
  cplx2reim62/2 -> t49/1
  Selector40/1 -> reim2cplx20/2
  in4_repeat1/1 -> rd_03/1
  cplx2reim62/1 -> t48/1
  Selector14/1 -> reim2cplx7/2
  Selector79/1 -> reim2cplx39/1
  Selector10/1 -> reim2cplx5/2
  dtc33/1 -> rd_30/1
  t87/1 -> Selector57/1
  cplx2reim5/1 -> rd_85/1
  t44/1 -> cplx2reim61/1
  cplx2reim59/1 -> t39/1
  Selector24/1 -> reim2cplx12/2
  t121/1 -> Selector78/1
  rd_79/1 -> adder8/2
  cplx2reim58/1 -> t36/1
  adder7/1 -> dtc7/1
  Selector71/1 -> reim2cplx35/1
  cplx2reim56/2 -> t31/1
  adder40/1 -> dtc40/1
  t108/1 -> Selector71/1
  crp_out_delay1/1 -> Delay6/1
  t29/1 -> cplx2reim56/1
  t145/1 -> Selector94/1
  t23/1 -> cplx2reim54/1
  cplx2reim52/2 -> t19/1
  adder31/1 -> dtc31/1
  adder36/1 -> dtc36/1
  cplx2reim52/1 -> t18/1
  cplx2reim51/2 -> t16/1
  Selector54/1 -> reim2cplx27/2
  Selector18/1 -> reim2cplx9/2
  dtc22/1 -> rd_52/1
  t14/1 -> cplx2reim51/1
  adder28/1 -> dtc28/1
  adder5/1 -> dtc5/1
  cplx2reim50/2 -> t13/1
  Selector95/1 -> reim2cplx47/1
  Selector74/1 -> reim2cplx37/2
  ValidRT_outrepeat/1 -> crp_out_delay2/1
  t111/1 -> Selector73/1
  cplx2reim47/1 -> adder47/2
  Selector5/1 -> reim2cplx2/1
  t142/1 -> Selector92/1
  rd_33/1 -> adder31/2
  t75/1 -> Selector49/1
  Selector93/1 -> reim2cplx46/1
  t79/1 -> Selector50/1
  Constant/1 -> Max1_stage1/2
  t141/1 -> Selector93/1
  t139/1 -> Selector90/1
  dtc45/1 -> rd_6/1
  Delay1_absorbed1/1 -> in4_repeat/1, Delay1_absorbed3/1, in3_repeat2/1
  t3/1 -> Selector1/1
  Selector88/1 -> reim2cplx44/2
  rd_57/1 -> adder19/2
  dtc40/1 -> rd_16/1
  dtc44/1 -> rd_8/1
  compare1/1 -> rd_510/1, rd_210/1
  Zero/1 -> Real-Imag to Complex/1, Real-Imag to Complex/2
  Selector83/1 -> reim2cplx41/1
  Selector13/1 -> reim2cplx6/1
  t126/1 -> Selector83/1
  rd_73/1 -> adder11/2
  Zero1/1 -> Real-Imag to Complex1/1, Real-Imag to Complex1/2
  Selector78/1 -> reim2cplx39/2
  adder39/1 -> dtc39/1
  t117/1 -> Selector77/1
  Selector47/1 -> reim2cplx23/1
  dtc38/1 -> rd_20/1
  Selector75/1 -> reim2cplx37/1
  dtc37/1 -> rd_22/1
  t99/1 -> Selector65/1
  Selector73/1 -> reim2cplx36/1
  rd_27/1 -> adder34/2
  reim2cplx2/1 -> cplx2reim2/1
  dtc36/1 -> rd_24/1
  rd_15/1 -> adder40/2
  dtc35/1 -> rd_26/1
  adder1/1 -> dtc1/1
  Selector66/1 -> reim2cplx33/2
  delayMatch3/1 -> Bus Creator2/1  "valid"
  adder32/1 -> dtc32/1
  t97/1 -> Selector62/1
  t94/1 -> Selector60/1
  t93/1 -> Selector61/1
  in3_repeat1/1 -> delayMatch4/1
  Selector8/1 -> reim2cplx4/2
  t88/1 -> Selector56/1
  Selector56/1 -> reim2cplx28/2
  adder27/1 -> dtc27/1
  Delay_absorbed/1 -> in0_repeat/1
  t64/1 -> Selector40/1
  t84/1 -> Selector55/1
  adder26/1 -> dtc26/1
  Selector53/1 -> reim2cplx26/1
  dtc26/1 -> rd_44/1
  Selector49/1 -> reim2cplx24/1
  t76/1 -> Selector48/1
  dtc/1 -> HwModeRegister/1
  t72/1 -> Selector47/1
  rd_102/1 -> switchEnable/3
  Selector46/1 -> reim2cplx23/2
  rd_712/1 -> Delay_Switch/1
  Delay11/1 -> Delay1_absorbed1/1
  Selector45/1 -> reim2cplx22/1
  reim2cplx36/1 -> cplx2reim36/1
  adder22/1 -> dtc22/1
  t69/1 -> Selector45/1
  Selector44/1 -> reim2cplx22/2
  PipelineRegister1/1 -> DataRT_outrepeat/1
  t67/1 -> Selector42/1
  reim2cplx3/1 -> cplx2reim3/1
  t66/1 -> Selector43/1
  Selector42/1 -> reim2cplx21/2
  dtc21/1 -> rd_54/1
  dtc20/1 -> rd_56/1
  in2_repeat3/1 -> rd_103/1
  reim2cplx14/1 -> cplx2reim14/1
  adder19/1 -> dtc19/1
  t60/1 -> Selector39/1
  adder18/1 -> dtc18/1
  in1_repeat/1 -> rd_811/1
  t58/1 -> Selector36/1
  dtc18/1 -> rd_60/1
  t55/1 -> Selector34/1
  dtc16/1 -> rd_64/1
  in2_repeat2/1 -> rd_111/1, rd_101/1
  t49/1 -> Selector30/1
  dtc15/1 -> rd_66/1
  t46/1 -> Selector28/1
  adder13/1 -> dtc13/1
  t43/1 -> Selector26/1
  adder12/1 -> dtc12/1
  t40/1 -> Selector24/1
  t39/1 -> Selector25/1
  cplx2reim8/1 -> rd_79/1
  Delay/1 -> Delay_absorbed/1
  t37/1 -> Selector22/1
  Selector22/1 -> reim2cplx11/2
  dtc11/1 -> rd_74/1
  adder10/1 -> dtc10/1
  Selector21/1 -> reim2cplx10/1
  t34/1 -> Selector20/1
  rd_17/1 -> adder39/2
  Selector20/1 -> reim2cplx10/2
  dtc10/1 -> rd_76/1
  adder9/1 -> dtc9/1
  t31/1 -> Selector18/1
  cplx2reim35/1 -> rd_25/1
  delayMatch2/1 -> ValidRT/1
  dtc9/1 -> rd_78/1
  crp_out_delay2/1 -> Delay3/1
  cplx2reim42/1 -> rd_11/1
  reim2cplx13/1 -> cplx2reim13/1
  dtc7/1 -> rd_82/1
  reim2cplx37/1 -> cplx2reim37/1
  Selector12/1 -> reim2cplx6/2
  dtc6/1 -> rd_84/1
  t18/1 -> Selector11/1
  Selector9/1 -> reim2cplx4/1
  dtc4/1 -> rd_88/1
  Selector6/1 -> reim2cplx3/2
  reim2cplx42/1 -> cplx2reim42/1
  dtc3/1 -> rd_90/1
  adder2/1 -> dtc2/1
  t10/1 -> Selector4/1
  t7/1 -> Selector2/1
  ValidResetCounter/1 -> ValidResetCounter_absorbed/1
  t6/1 -> Selector3/1
  dtc1/1 -> rd_94/1
  adder/1 -> dtc/1
  t1/1 -> crp_out_delay/1
  in3_repeat2/1 -> streaming_partition_streamed2/2(in1)
  in0_repeat/1 -> rd_110/1
  crp_out_delay8/1 -> HDL Counter/1
  DataMem/1 -> DataMem_absorbed/1
  in5_repeat/1 -> rd_411/1
  crp_out_delay11/1 -> ValidMem_lowered/1
  in3_repeat/1 -> delayMatch/1
  Delay5/1 -> Delay5_absorbed/1
  Delay4/1 -> Delay4_absorbed/1
  in1_repeat1/1 -> streaming_partition_streamed/1(in0)
  Delay1_absorbed3/1 -> in3_repeat/1
  rd_55/1 -> adder20/2
  valid_in/1 -> in1_repeat2/1
  reim2cplx8/1 -> cplx2reim8/1
  Row2Col_in1/1 -> streaming_partition_streamed1/1(in0)
  reim2cplx39/1 -> cplx2reim39/1
  in4_repeat/1 -> rd_311/1
  reim2cplx30/1 -> cplx2reim30/1
  t149/1 -> streaming_partition_streamed3/1(in0)
  rd_711/1 -> switchEnable/2
  cplx2reim34/1 -> rd_27/1
  reim2cplx9/1 -> cplx2reim9/1
  cplx2reim17/1 -> rd_61/1
  in0_repeat2/1 -> rd_0/1
  reim2cplx1/1 -> cplx2reim1/1
  rd_75/1 -> adder10/2
  reim2cplx6/1 -> cplx2reim6/1
  reim2cplx10/1 -> cplx2reim10/1
  reim2cplx11/1 -> cplx2reim11/1
  rd_29/1 -> adder33/2
  reim2cplx15/1 -> cplx2reim15/1
  reim2cplx46/1 -> cplx2reim46/1
  reim2cplx45/1 -> cplx2reim45/1
  cplx2reim25/1 -> rd_45/1
  reim2cplx40/1 -> cplx2reim40/1
  reim2cplx19/1 -> cplx2reim19/1
  reim2cplx44/1 -> cplx2reim44/1
  reim2cplx35/1 -> cplx2reim35/1
  cplx2reim14/1 -> rd_67/1
  rd_77/1 -> adder9/2
  reim2cplx21/1 -> cplx2reim21/1
  reim2cplx22/1 -> cplx2reim22/1
  reim2cplx23/1 -> cplx2reim23/1
  reim2cplx38/1 -> cplx2reim38/1
  reim2cplx25/1 -> cplx2reim25/1
  rd_65/1 -> adder15/2
  reim2cplx27/1 -> cplx2reim27/1
  cplx2reim18/1 -> rd_59/1
  reim2cplx28/1 -> cplx2reim28/1
  reim2cplx29/1 -> cplx2reim29/1
  rd_91/1 -> adder2/2
  reim2cplx31/1 -> cplx2reim31/1
  reim2cplx34/1 -> cplx2reim34/1
  reim2cplx41/1 -> cplx2reim41/1
  reim2cplx5/1 -> cplx2reim5/1
  Delay4_absorbed/1 -> in0_repeat2/1
  rd_7/1 -> adder44/2
  cplx2reim40/1 -> rd_15/1
  cplx2reim39/1 -> rd_17/1
  rd_43/1 -> adder26/2
  cplx2reim36/1 -> rd_23/1
  rd_11/1 -> adder42/2
  rd_13/1 -> adder41/2
  rd_69/1 -> adder13/2
  cplx2reim33/1 -> rd_29/1
  cplx2reim30/1 -> rd_35/1
  cplx2reim19/1 -> rd_57/1
  rd_21/1 -> adder37/2
  rd_25/1 -> adder35/2
  rd_35/1 -> adder30/2
  cplx2reim24/1 -> rd_47/1
  cplx2reim22/1 -> rd_51/1
  rd_81/1 -> adder7/2
  cplx2reim21/1 -> rd_53/1
  rd_37/1 -> adder29/2
  rd_39/1 -> adder28/2
  rd_41/1 -> adder27/2
  cplx2reim16/1 -> rd_63/1
  rd_47/1 -> adder24/2
  cplx2reim15/1 -> rd_65/1
  rd_53/1 -> adder21/2
  cplx2reim13/1 -> rd_69/1
  cplx2reim12/1 -> rd_71/1
  cplx2reim10/1 -> rd_75/1
  rd_59/1 -> adder18/2
  cplx2reim9/1 -> rd_77/1
  rd_63/1 -> adder16/2
  cplx2reim7/1 -> rd_81/1
  cplx2reim6/1 -> rd_83/1
  cplx2reim4/1 -> rd_87/1
  cplx2reim3/1 -> rd_89/1
  rd_0/1 -> t/1
  cplx2reim1/1 -> rd_93/1
  rd_87/1 -> adder4/2
  rd_95/1 -> adder/2
  rd_93/1 -> adder1/2
  rd_49/1 -> adder23/2
  rd_210/1 -> switch/2
  rd_310/1 -> switch/3
  streaming_partition_streamed2/1(out0) -> t148/1
  streaming_partition_streamed3/1(out0) -> t151/1
